simulink model "Resistive_Model_1_our_data"  (R2020a)
settings: Solver=VariableStepAuto  StartTime=0.0  StopTime=10  RelTol=1e-3
libraries: powerlib x5
settings Model: Creator=mitch  LastModifiedBy=mitch

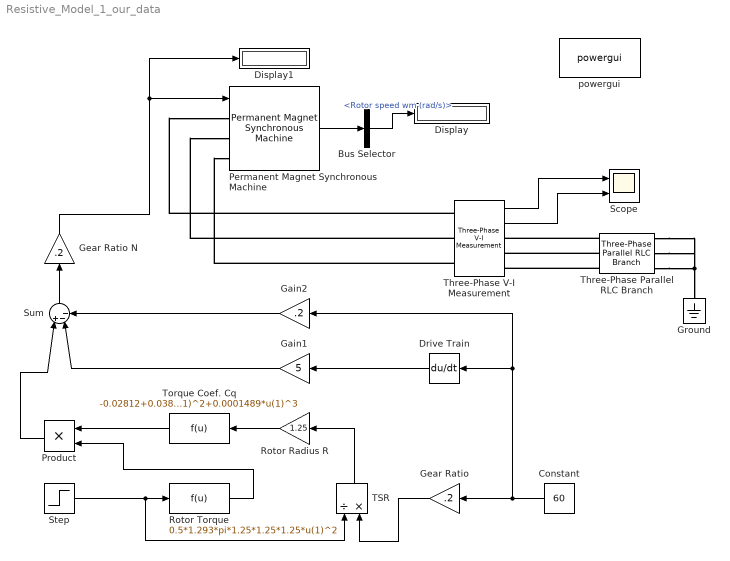
== system Resistive_Model_1_our_data ==
  Bus Selector : BusSelector  OutputSignals=Rotor speed wm (rad/s)
  Constant : Constant  Value=60
  Display : Display
  Display1 : Display
  Drive Train : Derivative
  Gain1 : Gain  Gain=5
  Gain2 : Gain  Gain=.2
  Gear Ratio : Gain  Gain=.2
  Gear Ratio N : Gain  Gain=.2
  Ground : powerlib/Elements/Ground  LConnTagsString=a
  Permanent Magnet Synchronous Machine : powerlib/Machines/Permanent Magnet Synchronous Machine  NbPhases=3  FluxDistribution=Sinusoidal  RotorType=Round  MechanicalLoad=Torque Tm  PresetModel="01:  0.8 Nm 300 Vdc 3000 RPM - 0.8 Nm"  ShowDetailedParameters=on  MeasurementBus=off  Resistance=18.7  Inductance=8.5e-3  dqInductances=[8.5e-3,8.5e-3]  La=0.02682  MachineConstant=Flux linkage established by magnets (V.s)  Flux=0.1716  VoltageCst=62.2496  TorqueCst=0.5148  Flat=120  Mechanical=[2.26e-05 1.349e-05 2 0]  PolePairs=2  InitialConditions=[70,0, 3,3]  InitialConditions5ph=[0 0 0 0 0 0]  RefAngle=90 degrees behind phase A axis (modified Park)  IterativeDiscreteModel=Trapezoidal non iterative  TsBlock=-1  TsPowergui=0
  Product : Product
  Rotor Radius R : Gain  Gain=1.25
  Rotor Torque : Fcn  Expr=0.5*1.293*pi*1.25*1.25*1.25*u(1)^2
  Scope : Scope  NumInputPorts=2
  Step : Step  Before=4  After=8  SampleTime=0
  Sum : Sum  Inputs=|+--
  "TSR " : Product  Inputs=/*
  Three-Phase Parallel RLC Branch : powerlib/Elements/Three-Phase Parallel RLC Branch  LConnTagsString=A|B|C  RConnTagsString=A|B|C  BranchType=R  Resistance=10  Inductance=1e-3  Capacitance=1e-6  Measurements=None
      settings: SourceProductBaseCode=PS
  Three-Phase V-I Measurement : powerlib/Measurements/Three-Phase V-I Measurement  VoltageMeasurement=phase-to-ground  SetLabelV=off  LabelV=Vabc  Vpu=off  VpuLL=off  CurrentMeasurement=yes  SetLabelI=off  LabelI=Iabc  Ipu=off  Pbase=100e6  Vbase=500e3  OutputType=Complex  PhasorSimulation=off  PSBequivalent=0
  Torque Coef. Cq : Fcn  Expr=-0.02812+0.038576*u(1)-0.0045912*u(1)^2+0.0001489*u(1)^3
  powergui : powerlib/powergui  Priority=1  SimulationMode=Discrete  SampleTime=5e-05  frequency=60  Iterations=50  frequencyindice=0  Pbase=100e6  ErrMax=1e-4  UnitsV=kV  UnitsW=MW  buscounter=0  FunctionMessages=off  echomessages=off  EnableUseOfTLC=off  CurrentSourceSwitches=off  DisableSnubberDevices=off  DisableRonSwitches=off  DisableVfSwitches=off  DisplayEquations=off  AutomaticDiscreteSolvers=off  SolverType=Tustin/Backward Euler (TBE)  Interpol=off  ExternalGateDelay=off  methode=off  Ts=100  x0status=blocks  SPID=on  SwTol=0  HookPort=off  NonlinearTolerance=1e-4  nMaxIteration=100  ContinueOnMaxIteration=off  RestoreLinks=warning  ResistiveCurrentMeasurement=off  Frange=[0:2:500]  Ylog=off  Xlog=on  ShowGrid=off  save=off  variable=ZData  structure=0  ZoomFFT=off  StartTime=0.0  cycles=1  DisplayStyle=1  fundamental=60  FreqAxis=off  MaxFrequency=1000  frequencyindicesteady=1  RmsSteady=1  display=off
  wires:
  Step/1 -> "TSR "/1, Rotor Torque/1
  Rotor Torque/1 -> Product/2
  Torque Coef. Cq/1 -> Product/1
  Rotor Radius R/1 -> Torque Coef. Cq/1
  Constant/1 -> Gain2/1, Drive Train/1, Gear Ratio/1
  Drive Train/1 -> Gain1/1
  Product/1 -> Sum/1
  Gain1/1 -> Sum/2
  Gain2/1 -> Sum/3
  Gear Ratio N/1 -> Display1/1, Permanent Magnet Synchronous Machine/1
  Sum/1 -> Gear Ratio N/1
  Three-Phase V-I Measurement/2 -> Scope/2
  Three-Phase V-I Measurement/1 -> Scope/1
  Permanent Magnet Synchronous Machine/1 -> Bus Selector/1
  Bus Selector/1 -> Display/1  "<Rotor speed wm (rad/s)>"
  Gear Ratio/1 -> "TSR "/2
  "TSR "/1 -> Rotor Radius R/1
  connections:
  Three-Phase V-I Measurement/LConn3 -- Permanent Magnet Synchronous Machine/LConn3
  Three-Phase V-I Measurement/LConn2 -- Permanent Magnet Synchronous Machine/LConn2
  Three-Phase V-I Measurement/LConn1 -- Permanent Magnet Synchronous Machine/LConn1
  Three-Phase Parallel RLC Branch/LConn1 -- Three-Phase V-I Measurement/RConn1
  Three-Phase Parallel RLC Branch/LConn2 -- Three-Phase V-I Measurement/RConn2
  Three-Phase Parallel RLC Branch/LConn3 -- Three-Phase V-I Measurement/RConn3
  Three-Phase Parallel RLC Branch/RConn1 -- Three-Phase Parallel RLC Branch/RConn2 -- Three-Phase Parallel RLC Branch/RConn3 -- Ground/LConn1
